simulink model "VOOtest"  (R2023b)
settings: Solver=FixedStepAuto  StartTime=0.0  StopTime=10.0  FixedStep=1e-3  RelTol=1e-3  EnableMultiTasking=on
settings Model: ExtModeTrigDuration=5  Creator=mathewgaluszka  LastModifiedBy=mathewgaluszka
settings OptimizationCC: EnhancedBackFolding=on  PassReuseOutputArgsAs=Individual arguments  ZeroExternalMemoryAtStartup=off  ZeroInternalMemoryAtStartup=off  MaxStackSize=64  OptimizeBlockOrder=speed  DifferentSizesBufferReuse=on  OptimizationCustomize=off  EfficientTunableParamExpr=on
settings DebuggingCC: ParameterTunabilityLossMsg=error
settings HardwareCC: ProdBitPerPointer=32  ProdBitPerSizeT=32  ProdBitPerPtrDiffT=32  ProdLargestAtomicInteger=Long  ProdLargestAtomicFloat=Double  ProdWordSize=32  ProdHWDeviceType=ARM Compatible->ARM Cortex
settings SFSimCC: MATLABDynamicMemAlloc=off
settings RTWCC: Description=Embedded Coder  SystemTargetFile=ert.tlc  HardwareBoard=NXP FRDM-K64F  TLCOptions="-aInlineSetEventsForThisBaseRateFcn=TLC_FALSE -aSuppressMultiTaskScheduler=TLC_FALSE  -aRateBasedStepFcn=0"  TemplateMakefile=ert_default_tmf  Toolchain=GNU Tools for ARM Embedded Processors
settings CodeAppCC: ForceParamTrailComments=on  IgnoreCustomStorageClasses=off  OperatorAnnotations=on  SimulinkDataObjDesc=on  SFDataObjDesc=on  InsertBlockDesc=on
settings ERTTargetCC: ExtModeTransport=4  ExtModeMexFile=sendToCommService

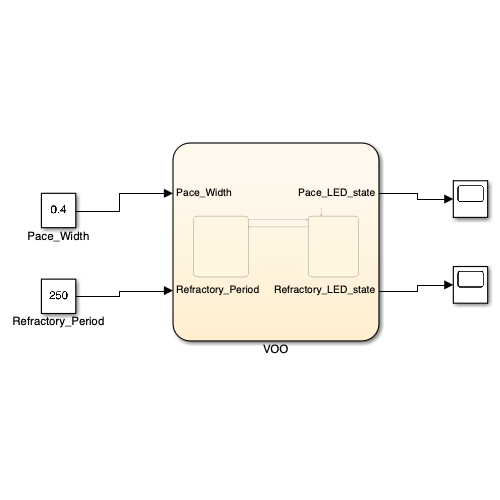
[thumbnail: Simulink's stored preview of the top-level diagram]
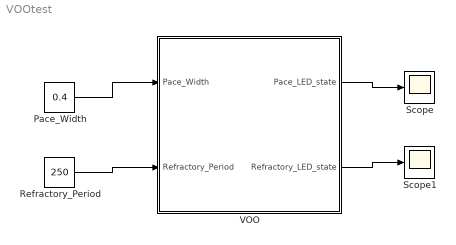
== system VOOtest ==
  Pace_Width : Constant  Value=0.4
  Refractory_Period : Constant  Value=250
  Scope : Scope
  Scope1 : Scope
  VOO : Stateflow chart  TreatAsAtomicUnit=on
  wires:
  Pace_Width/1 -> VOO/1(Pace_Width)
  Refractory_Period/1 -> VOO/2(Refractory_Period)
  VOO/1(Pace_LED_state) -> Scope/1
  VOO/2(Refractory_LED_state) -> Scope1/1

== stateflow chart VOOtest/VOO ==
  state Pace
    entry:
    Pace_LED_state=true;
    Refractory_LED_state=false;
    D2_PACE_CHARGE_CTRL=0;
    D10_PACE_GND_CTRL=1;
    D8_ATR_PACE_CTRL=0;
    D11_ATR_GND_CTRL=0;
    D4_Z_ATR_CTRL=0;
    D7_Z_VENT_CTRL=0;
    D12_VENT_GND_CTRL=0;
    D9_VENT_PACE_CTRL=1;
  state Refractory
    entry:
    Pace_LED_state=false;
    Refractory_LED_state=true;
    D10_PACE_GND_CTRL=1;
    D9_VENT_PACE_CTRL=0;
    D4_Z_ATR_CTRL=0;
    D7_Z_VENT_CTRL=0;
    D8_ATR_PACE_CTRL=0;
    D11_ATR_GND_CTRL=0;
    D12_VENT_GND_CTRL=1;
    D2_PACE_CHARGE_CTRL=1;
  (default) -> Refractory
  Pace -> Refractory : [after(Pace_Width,msec)]
  Refractory -> Pace : [after(Refractory_Period,msec)]
  data: Pace_Width input; Refractory_Period input; Pace_LED_state output; Refractory_LED_state output
